simulink model "DigitalTwin_v8"  (R2023a)
settings: Solver=ode23t  StartTime=0.0  StopTime=600  RelTol=1e-3  AbsTol=1e-3
model workspace: external: MATLAB File C:\Users\claud\OneDrive - TUM\COME -TUM\Software lab\Three_wheeled_base\simscape_1\Three_wheeled_base_DataFile1.m (data not in the file)
values from neighbouring files (symbols this model uses):
  brick_pick_global_xy = [brick_pick_global_xy, new_column]    [Three_wheeled_base_DataFile2.m]
  brick_place_global_xy = [brick_place_global_xy, new_column]    [Three_wheeled_base_DataFile2.m]
  platform_destination_mat = [ 1.0 0; 5 0; 0 0; 0 5 ... (first row only)    [Three_wheeled_base_DataFile2.m]
  robotData =     [points_on_pad.mat]
  smiData =     [points_on_pad.mat]    (also in road_points_on_pad.mat)
undefined symbols (not defined in the file or in its folder): X, Y, Z
libraries: sm_lib x246, nesl_utility x86, fl_lib x12, batteryecm_lib x5, ee_lib x3, robotcorelib x1, robotalgslib x1
(part 2 of 8)

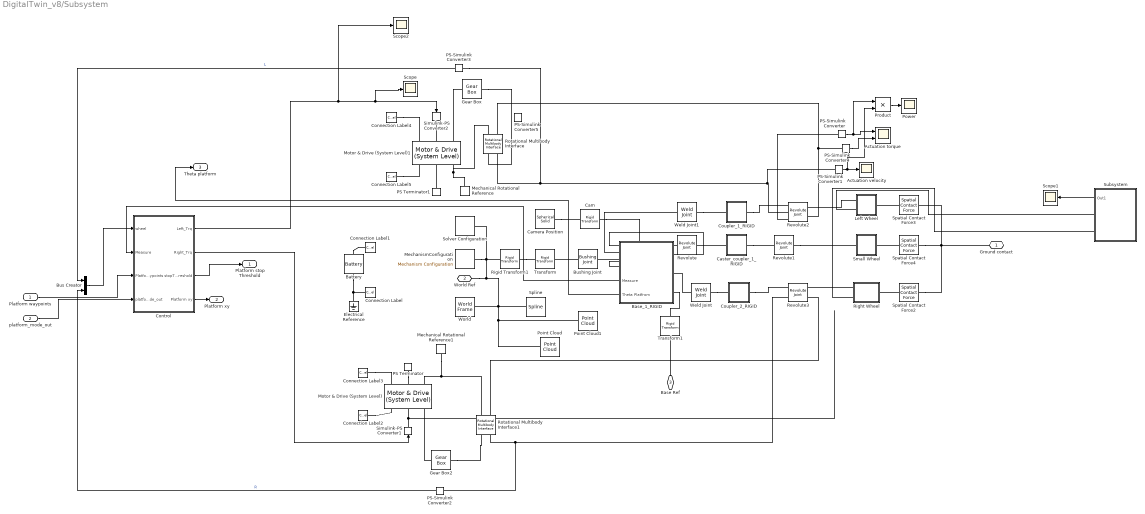
== system DigitalTwin_v8/Subsystem ==
  Platform waypoints : Inport
  platform_mode_out : Inport  Port=2
  Actuation torque : Scope  NumInputPorts=2
  Actuation velocity : Scope
  Base_1_RIGID : Subsystem
      settings: PortSchema="{\"entries\":[{\"content\":{\"sides\":[{\"content\":{\"connectorIds\":[\"LConn1\",\"LConn2\",\"Out1\",\"Out2\"]},\"type\":\"ConnectorPlacement.EquallySpacedRectSide\",\"uuid\":\"915af11b-fe8a-4d36-b5cd-ea91b8047f29\"},{\"content\":{\"connectorIds\":[\"RConn1\",\"RConn2\",\"RConn3\"],\"side\":\"RIGHT\"},\"type\":\"ConnectorPlacement.EquallySpacedRectSide\",\"uuid\":\"f3343107-e0e0-4658-8996-ee38c7783267\"},{\"content\":{\"side\":\"TOP\"},\"type\":\"ConnectorPlacement.EquallySpacedRectSide\",\"uuid\":\"4328f01d-baa2-48a9-97ea-3cbc7b3f5381\"}]},\"type\":\"ConnectorPlacement.EquallySpacedConnector\",\"uuid\":\"91d1c2c9-868d-4769-9f96-4594451c2c0c\"}],\"packageUris\":[\"http://schema.mathworks.com/mf0/Connector/R2020b\"],\"version\":\"1.0\"}"
  Battery : batteryecm_lib/Battery  Vnom=12 V  prm_dir=simscape.enum.battery.prm_dir.disabled  R1_dis=2 Ohm  R1_ch=2 Ohm  R1=2 Ohm  prm_AH=simscape.enum.battery.prm_AH.infinite  AH=50 A*hr  V1=11.5 V  AH1=25 A*hr  prm_R2=simscape.enum.battery.prm_R2.disabled  R2=2000 Ohm  Tmeas=298.15 K  charge_measurement_port=simscape.enum.battery.enable.no  prm_dyn=simscape.enum.battery.prm_dyn.off  Rp1=0.005 Ohm  tau1=30 s  Rp2=0.005 Ohm  tau2=30 s  Rp3=0.005 Ohm  tau3=30 s  Rp4=0.005 Ohm  tau4=30 s  Rp5=0.005 Ohm  tau5=30 s  prm_fade=simscape.enum.battery.prm_fade.disabled  N_fade=100  AH_fade=45 A*hr  R1_fade=2.02 Ohm  R1_ch_fade=2.02 Ohm  V1_fade=10.35 V  prm_age=simscape.enum.battery.prm_age.disabled  prm_age_OCV=simscape.enum.battery.prm_age_OCV.OCV  OCV_age=0.9  SOC_age=60  Tmeas_age=298.15 K  delta_time_age_vec=[0] d  temperature_age_vec=[273] K  OCV_scaling_age=2.2134e6  OCV_offset_age=1.632e6  temp_exp_age=0.515833569 V  t_exp_age=0.75  Vnom_T2=12 V  R1_T2=2.2 Ohm  R1_T2_dis=2.2 Ohm  R1_T2_ch=2.2 Ohm  V1_T2=11.4 V  R2_T2=2200 Ohm  Rp1_T2=0.005 Ohm  tau1_T2=30 s  Rp2_T2=0.005 Ohm  tau2_T2=30 s  Rp3_T2=0.005 Ohm  tau3_T2=30 s  Rp4_T2=0.005 Ohm  tau4_T2=30 s  Rp5_T2=0.005 Ohm  tau5_T2=30 s  Tmeas2=273.15 K  thermal_port=simscape.enum.thermaleffects.omit  thermal_mass=30000 J/K  i_specify=off  i_priority=None  i=0 A  i_nominal_specify=off  i_nominal_unit=A  i_nominal_value=1  v_specify=off  v_priority=None  v=0 V  v_nominal_specify=off  v_nominal_unit=V  v_nominal_value=1  charge_specify=off  charge_priority=High  charge=50 A*hr  charge_nominal_specify=off  charge_nominal_unit=A*hr  charge_nominal_value=1  num_cycles_specify=off  num_cycles_priority=High  num_cycles=0  num_cycles_nominal_specify=off  num_cycles_nominal_unit=1  num_cycles_nominal_value=1  temperature_specify=off  temperature_priority=High  temperature=298.15 K  temperature_nominal_specify=off  temperature_nominal_unit=K  temperature_nominal_value=1
  Bus Creator : BusCreator  Inputs=2
  Bushing Joint : sm_lib/Joints/Bushing Joint  JointMode=Normal  SenseConstraintForce=off  SenseConstraintForceX=off  SenseConstraintForceY=off  SenseConstraintForceZ=off  SenseConstraintTorque=off  SenseConstraintTorqueX=off  SenseConstraintTorqueY=off  SenseConstraintTorqueZ=off  SenseTotalForce=off  SenseTotalForceX=off  SenseTotalForceY=off  SenseTotalForceZ=off  SenseTotalTorque=off  SenseTotalTorqueX=off  SenseTotalTorqueY=off  SenseTotalTorqueZ=off  CompositeWrenchDir=FollowerOnBase  CompositeWrenchFrame=BaseFrame  PxEquilibriumPosition=0  PxEquilibriumPositionUnits=m  PxSpringStiffness=0  PxSpringStiffnessUnits=N/m  PxDampingCoefficient=0  PxDampingCoefficientUnits=N/(m/s)  PxTorqueActuationMode=NoTorque  PxMotionActuationMode=ComputedMotion  PxSensePosition=off  PxSenseVelocity=off  PxSenseAcceleration=off  PxSenseTorqueForce=off  PxSenseLowerLimitTorqueForce=off  PxSenseUpperLimitTorqueForce=off  PxLowerLimitSpecify=off  PxLowerLimitBound=-1  PxLowerLimitBoundUnits=m  PxLowerLimitStiffness=1e6  PxLowerLimitStiffnessUnits=N/m  PxLowerLimitDamping=1e3  PxLowerLimitDampingUnits=N/(m/s)  PxLowerLimitTransitionRegionWidth=1e-4  PxLowerLimitTransitionRegionWidthUnits=m  PxUpperLimitSpecify=off  PxUpperLimitBound=1  PxUpperLimitBoundUnits=m  PxUpperLimitStiffness=1e6  PxUpperLimitStiffnessUnits=N/m  PxUpperLimitDamping=1e3  PxUpperLimitDampingUnits=N/(m/s)  PxUpperLimitTransitionRegionWidth=1e-4  PxUpperLimitTransitionRegionWidthUnits=m  PxPositionTargetSpecify=off  PxPositionTargetPriority=High  PxPositionTargetValue=0  PxPositionTargetValueUnits=m  PxVelocityTargetSpecify=off  PxVelocityTargetPriority=High  PxVelocityTargetValue=0  PxVelocityTargetValueUnits=m/s  PyEquilibriumPosition=0  PyEquilibriumPositionUnits=m  PySpringStiffness=0  PySpringStiffnessUnits=N/m  PyDampingCoefficient=0  PyDampingCoefficientUnits=N/(m/s)  PyTorqueActuationMode=NoTorque  PyMotionActuationMode=ComputedMotion  PySensePosition=off  PySenseVelocity=off  PySenseAcceleration=off  PySenseTorqueForce=off  PySenseLowerLimitTorqueForce=off  PySenseUpperLimitTorqueForce=off  PyLowerLimitSpecify=off  PyLowerLimitBound=-1  PyLowerLimitBoundUnits=m  PyLowerLimitStiffness=1e6  PyLowerLimitStiffnessUnits=N/m  PyLowerLimitDamping=1e3  PyLowerLimitDampingUnits=N/(m/s)  PyLowerLimitTransitionRegionWidth=1e-4  PyLowerLimitTransitionRegionWidthUnits=m  PyUpperLimitSpecify=off  PyUpperLimitBound=1  PyUpperLimitBoundUnits=m  PyUpperLimitStiffness=1e6  PyUpperLimitStiffnessUnits=N/m  PyUpperLimitDamping=1e3  PyUpperLimitDampingUnits=N/(m/s)  PyUpperLimitTransitionRegionWidth=1e-4  PyUpperLimitTransitionRegionWidthUnits=m  PyPositionTargetSpecify=off  PyPositionTargetPriority=High  PyPositionTargetValue=0  PyPositionTargetValueUnits=m  PyVelocityTargetSpecify=off  PyVelocityTargetPriority=High  PyVelocityTargetValue=0  PyVelocityTargetValueUnits=m/s  PzEquilibriumPosition=0  PzEquilibriumPositionUnits=m  PzSpringStiffness=0  PzSpringStiffnessUnits=N/m  PzDampingCoefficient=0  PzDampingCoefficientUnits=N/(m/s)  PzTorqueActuationMode=NoTorque  PzMotionActuationMode=ComputedMotion  PzSensePosition=off  PzSenseVelocity=off  PzSenseAcceleration=off  PzSenseTorqueForce=off  PzSenseLowerLimitTorqueForce=off  PzSenseUpperLimitTorqueForce=off  PzLowerLimitSpecify=off  PzLowerLimitBound=-1  PzLowerLimitBoundUnits=m  PzLowerLimitStiffness=1e6  PzLowerLimitStiffnessUnits=N/m  PzLowerLimitDamping=1e3  PzLowerLimitDampingUnits=N/(m/s)  PzLowerLimitTransitionRegionWidth=1e-4  PzLowerLimitTransitionRegionWidthUnits=m  PzUpperLimitSpecify=off  PzUpperLimitBound=1  PzUpperLimitBoundUnits=m  PzUpperLimitStiffness=1e6  PzUpperLimitStiffnessUnits=N/m  PzUpperLimitDamping=1e3  PzUpperLimitDampingUnits=N/(m/s)  PzUpperLimitTransitionRegionWidth=1e-4  PzUpperLimitTransitionRegionWidthUnits=m  PzPositionTargetSpecify=off  PzPositionTargetPriority=High  PzPositionTargetValue=0  PzPositionTargetValueUnits=m  PzVelocityTargetSpecify=off  PzVelocityTargetPriority=High  PzVelocityTargetValue=0  PzVelocityTargetValueUnits=m/s  RxEquilibriumPosition=0  RxEquilibriumPositionUnits=deg  RxSpringStiffness=0  RxSpringStiffnessUnits=N*m/deg  RxDampingCoefficient=0  RxDampingCoefficientUnits=N*m/(deg/s)  RxTorqueActuationMode=NoTorque  RxMotionActuationMode=ComputedMotion  RxSensePosition=off  RxSenseVelocity=off  RxSenseAcceleration=off  RxSenseTorqueForce=off  RxSenseLowerLimitTorqueForce=off  RxSenseUpperLimitTorqueForce=off  RxLowerLimitSpecify=off  RxLowerLimitBound=-90  RxLowerLimitBoundUnits=deg  RxLowerLimitStiffness=1e4  RxLowerLimitStiffnessUnits=N*m/deg  RxLowerLimitDamping=10  RxLowerLimitDampingUnits=N*m/(deg/s)  RxLowerLimitTransitionRegionWidth=0.1  RxLowerLimitTransitionRegionWidthUnits=deg  RxUpperLimitSpecify=off  RxUpperLimitBound=90  RxUpperLimitBoundUnits=deg  RxUpperLimitStiffness=1e4  RxUpperLimitStiffnessUnits=N*m/deg  RxUpperLimitDamping=10  RxUpperLimitDampingUnits=N*m/(deg/s)  RxUpperLimitTransitionRegionWidth=0.1  RxUpperLimitTransitionRegionWidthUnits=deg  RxPositionTargetSpecify=off  RxPositionTargetPriority=High  RxPositionTargetValue=0  RxPositionTargetValueUnits=deg  RxVelocityTargetSpecify=off  RxVelocityTargetPriority=High  RxVelocityTargetValue=0  RxVelocityTargetValueUnits=deg/s  RyEquilibriumPosition=0  RyEquilibriumPositionUnits=deg  RySpringStiffness=0  RySpringStiffnessUnits=N*m/deg  RyDampingCoefficient=0  RyDampingCoefficientUnits=N*m/(deg/s)  RyTorqueActuationMode=NoTorque  RyMotionActuationMode=ComputedMotion  RySensePosition=off  RySenseVelocity=off  RySenseAcceleration=off  RySenseTorqueForce=off  RySenseLowerLimitTorqueForce=off  RySenseUpperLimitTorqueForce=off  RyLowerLimitSpecify=off  RyLowerLimitBound=-90  RyLowerLimitBoundUnits=deg  RyLowerLimitStiffness=1e4  RyLowerLimitStiffnessUnits=N*m/deg  RyLowerLimitDamping=10  RyLowerLimitDampingUnits=N*m/(deg/s)  RyLowerLimitTransitionRegionWidth=0.1  RyLowerLimitTransitionRegionWidthUnits=deg  RyUpperLimitSpecify=off  RyUpperLimitBound=90  RyUpperLimitBoundUnits=deg  RyUpperLimitStiffness=1e4  RyUpperLimitStiffnessUnits=N*m/deg  RyUpperLimitDamping=10  RyUpperLimitDampingUnits=N*m/(deg/s)  RyUpperLimitTransitionRegionWidth=0.1  RyUpperLimitTransitionRegionWidthUnits=deg  RyPositionTargetSpecify=off  RyPositionTargetPriority=High  RyPositionTargetValue=0  RyPositionTargetValueUnits=deg  RyVelocityTargetSpecify=off  RyVelocityTargetPriority=High  RyVelocityTargetValue=0  RyVelocityTargetValueUnits=deg/s  RzEquilibriumPosition=0  RzEquilibriumPositionUnits=deg  RzSpringStiffness=0  RzSpringStiffnessUnits=N*m/deg  RzDampingCoefficient=0  RzDampingCoefficientUnits=N*m/(deg/s)  RzTorqueActuationMode=NoTorque  RzMotionActuationMode=ComputedMotion  RzSensePosition=off  RzSenseVelocity=off  RzSenseAcceleration=off  RzSenseTorqueForce=off  RzSenseLowerLimitTorqueForce=off  RzSenseUpperLimitTorqueForce=off  RzLowerLimitSpecify=off  RzLowerLimitBound=-90  RzLowerLimitBoundUnits=deg  RzLowerLimitStiffness=1e4  RzLowerLimitStiffnessUnits=N*m/deg  RzLowerLimitDamping=10  RzLowerLimitDampingUnits=N*m/(deg/s)  RzLowerLimitTransitionRegionWidth=0.1  RzLowerLimitTransitionRegionWidthUnits=deg  RzUpperLimitSpecify=off  RzUpperLimitBound=90  RzUpperLimitBoundUnits=deg  RzUpperLimitStiffness=1e4  RzUpperLimitStiffnessUnits=N*m/deg  RzUpperLimitDamping=10  RzUpperLimitDampingUnits=N*m/(deg/s)  RzUpperLimitTransitionRegionWidth=0.1  RzUpperLimitTransitionRegionWidthUnits=deg  RzPositionTargetSpecify=off  RzPositionTargetPriority=High  RzPositionTargetValue=0  RzPositionTargetValueUnits=deg  RzVelocityTargetSpecify=off  RzVelocityTargetPriority=High  RzVelocityTargetValue=0  RzVelocityTargetValueUnits=deg/s
  Cam : sm_lib/Frames and Transforms/Rigid Transform  TranslationMethod=Cartesian  TranslationStandardOffset=0  TranslationStandardOffsetUnits=m  TranslationStandardAxis=+Z  TranslationCartesianOffset=[1 1 1]  TranslationCartesianOffsetUnits=m  TranslationROffset=0  TranslationROffsetUnits=m  TranslationZOffset=0  TranslationZOffsetUnits=m  TranslationThetaOffset=0  TranslationThetaOffsetUnits=deg  RotationMethod=None  RotationAngleUnits=deg  RotationStandardAxis=+Z  RotationAngle=0.0  RotationArbitraryAxis=[0 0 1]  FollAlignAxisA=+X  BaseAlignAxisA=+Y  FollAlignAxisB=+Y  BaseAlignAxisB=+Z  RotationSequenceAxes=FollowerAxes  RotationSequence=XYX  RotationSequenceAngles=[0 0 0]  RotationSequenceAnglesUnits=deg  RotationMatrix=[1 0 0; 0 1 0; 0 0 1]  Quaternion=[1 0 0 0]
  Camera Position : sm_lib/Body Elements/Spherical Solid  GraphicAmbientColor=[0.15 0.15 0.15 1.0]  BasedOnType=Density  CenterOfMass=[0 0 0]  CenterOfMassUnits=m  GraphicDiffuseColor=[0.5 0.5 0.5]  Density=0  DensityUnits=kg/m^3  DoExposeReferenceFrame=on  GraphicEmissiveColor=[0.0 0.0 0.0 1.0]  ExportEntireGeometry=off  SerializedExposedGeometries=<ExposedGeometries/>  SerializedFrames=<Frames/>  MarkerShape=Sphere  MarkerSize=10  GraphicType=FromGeometry  InertiaType=CalculateFromGeometry  Mass=1  MassUnits=kg  MomentsOfInertia=[1 1 1]  MomentsOfInertiaUnits=kg*m^2  GraphicOpacity=1.0  ProductsOfInertia=[0 0 0]  ProductsOfInertiaUnits=kg*m^2  GraphicShininess=75  GraphicSpecularColor=[0.5 0.5 0.5 1.0]  SphereRadius=0.01  SphereRadiusUnits=m  GraphicVisPropType=SimpleVisualProperties
  Caster_coupler_1_RIGID : Subsystem
  Connection Label : ConnectionLabel  Label=N
  Connection Label1 : ConnectionLabel  Label=P
  Connection Label2 : ConnectionLabel  Label=P
  Connection Label3 : ConnectionLabel  Label=N
  Connection Label4 : ConnectionLabel  Label=P
  Connection Label5 : ConnectionLabel  Label=N
  Control : Subsystem
  Coupler_1_RIGID : Subsystem
  Coupler_2_RIGID : Subsystem
  Electrical Reference : fl_lib/Electrical/Electrical Elements/Electrical Reference
  Gear Box : fl_lib/Mechanical/Mechanisms/Gear Box  ratio=0.05*0+1  t_in_specify=off  t_in_priority=None  t_in=0 N*m  t_in_nominal_specify=off  t_in_nominal_unit=N*m  t_in_nominal_value=1  t_out_specify=off  t_out_priority=None  t_out=0 N*m  t_out_nominal_specify=off  t_out_nominal_unit=N*m  t_out_nominal_value=1
  Gear Box2 : fl_lib/Mechanical/Mechanisms/Gear Box  ratio=0.05*0+1  t_in_specify=off  t_in_priority=None  t_in=0 N*m  t_in_nominal_specify=off  t_in_nominal_unit=N*m  t_in_nominal_value=1  t_out_specify=off  t_out_priority=None  t_out=0 N*m  t_out_nominal_specify=off  t_out_nominal_unit=N*m  t_out_nominal_value=1
  Left Wheel : Subsystem
  Mechanical Rotational Reference : fl_lib/Mechanical/Rotational Elements/Mechanical Rotational Reference
  Mechanical Rotational Reference1 : fl_lib/Mechanical/Rotational Elements/Mechanical Rotational Reference
  MechanismConfiguration : sm_lib/Utilities/Mechanism Configuration  UniformGravity=Constant  GravityVector=[0 0 -9.80665]  GravityVectorUnits=m/s^2  LinearizationDelta=0.001  JointModeTransitionNonlinearIterations=2
  Motor & Drive (System Level) : ee_lib/Electromechanical/Motor & Drive (System Level)  torque_speed_param=ee.enum.electromech.envelope.tabulated  overtorque_param=ee.enum.electromech.overtorque.no  T_t=[.09, .08, .07, 0]*20 N*m  T_t_intermittent=[.36, .32, .28, 0] N*m  T_t_2D=[.09, .09, .09; .08, .08, .08; .07, .07, .07; 0, 0, 0] N*m  T_t_intermittent_2D=[.36, .36, .36; .32, .32, .32; .28, .28, .28; 0, 0, 0] N*m  w_t=[0, 3750, 7500, 8000] rpm  vdc_t=[6, 12, 24] V  torque_max=0.1 N*m  power_max=30 W  torque_max_intermittent=0.4 N*m  power_max_intermittent=120 W  time_overtorque=30 s  time_recover=60 s  Tc=0.02 s  losses_param=1  eff=100  w_eff=3750 rpm  T_eff=0.08 N*m  Piron=0 W  Pbase=0 W  w_eff_vec=[-8000, -4000, 0, 4000, 8000] rpm  T_eff_vec=[0, .03, .06, .09] N*m  v_eff_vec=[100, 250, 400] V  losses_mat=[1.49, 1.67, 2.21, 3.1; .42, .69, 1.14, 2.03; .06, .24, .78, 1.68; .42, .69, 1.14, 2.03; 1.49, 1.67, 2.21, 3.1] W  efficiency_mat=[95, 95, 95, 95; 95, 95, 95, 95; 95, 95, 95, 95; 95, 95, 95, 95; 95, 95, 95, 95]  losses_mat_3D=ones(5, 4, 3) W  efficiency_mat_3D=95 * ones(5, 4, 3)  Res=0 Ohm  enable_fault=simscape.enum.onoff.off  fault_condition=1  fault_threshold=0.5  J=5e-6 kg*m^2  lam=1e-5 N*m*s/rad  speed0=0 rpm  faulted_specify=off  faulted_priority=None  faulted=0  faulted_nominal_specify=off  faulted_nominal_unit=1  faulted_nominal_value=1  torqueLimitContinuous_specify=off  torqueLimitContinuous_priority=None  torqueLimitContinuous=0 N*m  torqueLimitContinuous_nominal_specify=off  torqueLimitContinuous_nominal_unit=N*m  torqueLimitContinuous_nominal_value=1  alpha=3.93e-3 1/K  Tmeas=25 degC  Tmeas2=125 degC  losses_mat_T2=[1.49, 1.74, 2.49, 3.74; .42, .67, 1.42, 2.67; .06, .31, 1.06, 2.31; .42, .67, 1.42, 2.67; 1.49, 1.74, 2.49, 3.74] W  efficiency_mat_T2=[95, 95, 95, 95; 95, 95, 95, 95; 95, 95, 95, 95; 95, 95, 95, 95; 95, 95, 95, 95]  losses_mat_3D_T2=ones(5, 4, 3) W  efficiency_mat_3D_T2=95 * ones(5, 4, 3)  thermal_mass=100 J/K  initial_temperature=25 degC
  Motor & Drive (System Level)1 : ee_lib/Electromechanical/Motor & Drive (System Level)  torque_speed_param=ee.enum.electromech.envelope.tabulated  overtorque_param=ee.enum.electromech.overtorque.no  T_t=[.09, .08, .07, 0]*20 N*m  T_t_intermittent=[.36, .32, .28, 0] N*m  T_t_2D=[.09, .09, .09; .08, .08, .08; .07, .07, .07; 0, 0, 0] N*m  T_t_intermittent_2D=[.36, .36, .36; .32, .32, .32; .28, .28, .28; 0, 0, 0] N*m  w_t=[0, 3750, 7500, 8000] rpm  vdc_t=[6, 12, 24] V  torque_max=0.1 N*m  power_max=30 W  torque_max_intermittent=0.4 N*m  power_max_intermittent=120 W  time_overtorque=30 s  time_recover=60 s  Tc=0.02 s  losses_param=1  eff=100  w_eff=3750 rpm  T_eff=0.08 N*m  Piron=0 W  Pbase=0 W  w_eff_vec=[-8000, -4000, 0, 4000, 8000] rpm  T_eff_vec=[0, .03, .06, .09] N*m  v_eff_vec=[100, 250, 400] V  losses_mat=[1.49, 1.67, 2.21, 3.1; .42, .69, 1.14, 2.03; .06, .24, .78, 1.68; .42, .69, 1.14, 2.03; 1.49, 1.67, 2.21, 3.1] W  efficiency_mat=[95, 95, 95, 95; 95, 95, 95, 95; 95, 95, 95, 95; 95, 95, 95, 95; 95, 95, 95, 95]  losses_mat_3D=ones(5, 4, 3) W  efficiency_mat_3D=95 * ones(5, 4, 3)  Res=0 Ohm  enable_fault=simscape.enum.onoff.off  fault_condition=1  fault_threshold=0.5  J=5e-6 kg*m^2  lam=1e-5 N*m*s/rad  speed0=0 rpm  faulted_specify=off  faulted_priority=None  faulted=0  faulted_nominal_specify=off  faulted_nominal_unit=1  faulted_nominal_value=1  torqueLimitContinuous_specify=off  torqueLimitContinuous_priority=None  torqueLimitContinuous=0 N*m  torqueLimitContinuous_nominal_specify=off  torqueLimitContinuous_nominal_unit=N*m  torqueLimitContinuous_nominal_value=1  alpha=3.93e-3 1/K  Tmeas=25 degC  Tmeas2=125 degC  losses_mat_T2=[1.49, 1.74, 2.49, 3.74; .42, .67, 1.42, 2.67; .06, .31, 1.06, 2.31; .42, .67, 1.42, 2.67; 1.49, 1.74, 2.49, 3.74] W  efficiency_mat_T2=[95, 95, 95, 95; 95, 95, 95, 95; 95, 95, 95, 95; 95, 95, 95, 95; 95, 95, 95, 95]  losses_mat_3D_T2=ones(5, 4, 3) W  efficiency_mat_3D_T2=95 * ones(5, 4, 3)  thermal_mass=100 J/K  initial_temperature=25 degC
      settings: LogSimulationData=on
  PS Terminator : fl_lib/Physical Signals/Sinks/PS Terminator
  PS Terminator1 : fl_lib/Physical Signals/Sinks/PS Terminator
  PS-Simulink Converter : nesl_utility/PS-Simulink Converter  PhysicalDomain=network_engine_domain  SubClassName=ps_output  LeftPortType=input  RightPortType=output  PseudoPeriodic=off  Frequencies=[]  VectorFormat=inherit  Unit=N*m  AffineConversion=off
  PS-Simulink Converter1 : nesl_utility/PS-Simulink Converter  PhysicalDomain=network_engine_domain  SubClassName=ps_output  LeftPortType=input  RightPortType=output  PseudoPeriodic=off  Frequencies=[]  VectorFormat=inherit  Unit=rad/s  AffineConversion=off
  PS-Simulink Converter2 : nesl_utility/PS-Simulink Converter  PhysicalDomain=network_engine_domain  SubClassName=ps_output  LeftPortType=input  RightPortType=output  PseudoPeriodic=off  Frequencies=[]  VectorFormat=inherit  Unit=inherit  AffineConversion=off
  PS-Simulink Converter3 : nesl_utility/PS-Simulink Converter  PhysicalDomain=network_engine_domain  SubClassName=ps_output  LeftPortType=input  RightPortType=output  PseudoPeriodic=off  Frequencies=[]  VectorFormat=inherit  Unit=inherit  AffineConversion=off
  PS-Simulink Converter4 : nesl_utility/PS-Simulink Converter  PhysicalDomain=network_engine_domain  SubClassName=ps_output  LeftPortType=input  RightPortType=output  PseudoPeriodic=off  Frequencies=[]  VectorFormat=inherit  Unit=N*m  AffineConversion=off
  PS-Simulink Converter5 : nesl_utility/PS-Simulink Converter  PhysicalDomain=network_engine_domain  SubClassName=ps_output  LeftPortType=input  RightPortType=output  PseudoPeriodic=off  Frequencies=[]  VectorFormat=inherit  Unit=inherit  AffineConversion=off
  Point Cloud : sm_lib/Curves and Surfaces/Point Cloud  CoordinatesMatrix=plotPoint_mtx  CoordinatesMatrixUnits=m  GraphicType=MarkerCloud  GraphicSphereRadius=1e-1  GraphicSphereRadiusUnits=m  GraphicVisPropType=SimpleVisualProperties  GraphicDiffuseColor=[1 0 1]  GraphicOpacity=1.0  GraphicSpecularColor=[0.5 0.5 0.5 1.0]  GraphicAmbientColor=[0.15 0.15 0.15 1.0]  GraphicEmissiveColor=[0.0 0.0 0.0 1.0]  GraphicShininess=75
  Point Cloud1 : sm_lib/Curves and Surfaces/Point Cloud  CoordinatesMatrix="[0.0253598785439431\t4.98644041888993\t1.45178955108506;-0.00960382399913822\t5.59952231514609\t0.175377640503004;-0.00940823618023848\t5.60012137569571\t0.399787372013566]"  CoordinatesMatrixUnits=m  GraphicType=MarkerCloud  GraphicSphereRadius=2.5e-2  GraphicSphereRadiusUnits=m  GraphicVisPropType=SimpleVisualProperties  GraphicDiffuseColor=[0.851 0.3255 0.09804]  GraphicOpacity=1.0  GraphicSpecularColor=[0.5 0.5 0.5 1.0]  GraphicAmbientColor=[0.15 0.15 0.15 1.0]  GraphicEmissiveColor=[0.0 0.0 0.0 1.0]  GraphicShininess=75
  Power : Scope
  Product : Product
  Revolute : sm_lib/Joints/Revolute Joint  JointMode=Normal  SenseConstraintForce=off  SenseConstraintForceX=off  SenseConstraintForceY=off  SenseConstraintForceZ=off  SenseConstraintTorque=off  SenseConstraintTorqueX=off  SenseConstraintTorqueY=off  SenseConstraintTorqueZ=off  SenseTotalForce=off  SenseTotalForceX=off  SenseTotalForceY=off  SenseTotalForceZ=off  SenseTotalTorque=off  SenseTotalTorqueX=off  SenseTotalTorqueY=off  SenseTotalTorqueZ=off  CompositeWrenchDir=FollowerOnBase  CompositeWrenchFrame=BaseFrame  EquilibriumPosition=0  EquilibriumPositionUnits=deg  SpringStiffness=0  SpringStiffnessUnits=N*m/deg  DampingCoefficient=0  DampingCoefficientUnits=N*m/(deg/s)  TorqueActuationMode=NoTorque  MotionActuationMode=ComputedMotion  SensePosition=off  SenseVelocity=off  SenseAcceleration=off  SenseTorqueForce=off  SenseLowerLimitTorqueForce=off  SenseUpperLimitTorqueForce=off  LowerLimitSpecify=off  LowerLimitBound=-90  LowerLimitBoundUnits=deg  LowerLimitStiffness=1e4  LowerLimitStiffnessUnits=N*m/deg  LowerLimitDamping=10  LowerLimitDampingUnits=N*m/(deg/s)  LowerLimitTransitionRegionWidth=0.1  LowerLimitTransitionRegionWidthUnits=deg  UpperLimitSpecify=off  UpperLimitBound=90  UpperLimitBoundUnits=deg  UpperLimitStiffness=1e4  UpperLimitStiffnessUnits=N*m/deg  UpperLimitDamping=10  UpperLimitDampingUnits=N*m/(deg/s)  UpperLimitTransitionRegionWidth=0.1  UpperLimitTransitionRegionWidthUnits=deg  PositionTargetSpecify=on  PositionTargetPriority=Low  PositionTargetValue=smiData.RevoluteJoint(1).Rz.Pos  PositionTargetValueUnits=deg  VelocityTargetSpecify=off  VelocityTargetPriority=High  VelocityTargetValue=0  VelocityTargetValueUnits=deg/s
  Revolute1 : sm_lib/Joints/Revolute Joint  JointMode=Normal  SenseConstraintForce=off  SenseConstraintForceX=off  SenseConstraintForceY=off  SenseConstraintForceZ=off  SenseConstraintTorque=off  SenseConstraintTorqueX=off  SenseConstraintTorqueY=off  SenseConstraintTorqueZ=off  SenseTotalForce=off  SenseTotalForceX=off  SenseTotalForceY=off  SenseTotalForceZ=off  SenseTotalTorque=off  SenseTotalTorqueX=off  SenseTotalTorqueY=off  SenseTotalTorqueZ=off  CompositeWrenchDir=FollowerOnBase  CompositeWrenchFrame=BaseFrame  EquilibriumPosition=0  EquilibriumPositionUnits=deg  SpringStiffness=0  SpringStiffnessUnits=N*m/deg  DampingCoefficient=0  DampingCoefficientUnits=N*m/(deg/s)  TorqueActuationMode=NoTorque  MotionActuationMode=ComputedMotion  SensePosition=off  SenseVelocity=off  SenseAcceleration=off  SenseTorqueForce=off  SenseLowerLimitTorqueForce=off  SenseUpperLimitTorqueForce=off  LowerLimitSpecify=off  LowerLimitBound=-90  LowerLimitBoundUnits=deg  LowerLimitStiffness=1e4  LowerLimitStiffnessUnits=N*m/deg  LowerLimitDamping=10  LowerLimitDampingUnits=N*m/(deg/s)  LowerLimitTransitionRegionWidth=0.1  LowerLimitTransitionRegionWidthUnits=deg  UpperLimitSpecify=off  UpperLimitBound=90  UpperLimitBoundUnits=deg  UpperLimitStiffness=1e4  UpperLimitStiffnessUnits=N*m/deg  UpperLimitDamping=10  UpperLimitDampingUnits=N*m/(deg/s)  UpperLimitTransitionRegionWidth=0.1  UpperLimitTransitionRegionWidthUnits=deg  PositionTargetSpecify=on  PositionTargetPriority=Low  PositionTargetValue=smiData.RevoluteJoint(2).Rz.Pos  PositionTargetValueUnits=deg  VelocityTargetSpecify=off  VelocityTargetPriority=High  VelocityTargetValue=0  VelocityTargetValueUnits=deg/s
  Revolute2 : sm_lib/Joints/Revolute Joint  JointMode=Normal  SenseConstraintForce=off  SenseConstraintForceX=off  SenseConstraintForceY=off  SenseConstraintForceZ=off  SenseConstraintTorque=off  SenseConstraintTorqueX=off  SenseConstraintTorqueY=off  SenseConstraintTorqueZ=off  SenseTotalForce=off  SenseTotalForceX=off  SenseTotalForceY=off  SenseTotalForceZ=off  SenseTotalTorque=off  SenseTotalTorqueX=off  SenseTotalTorqueY=off  SenseTotalTorqueZ=off  CompositeWrenchDir=FollowerOnBase  CompositeWrenchFrame=BaseFrame  EquilibriumPosition=0  EquilibriumPositionUnits=deg  SpringStiffness=0  SpringStiffnessUnits=N*m/deg  DampingCoefficient=0.001  DampingCoefficientUnits=N*m/(deg/s)  TorqueActuationMode=InputTorque  MotionActuationMode=ComputedMotion  SensePosition=off  SenseVelocity=on  SenseAcceleration=off  SenseTorqueForce=on  SenseLowerLimitTorqueForce=off  SenseUpperLimitTorqueForce=off  LowerLimitSpecify=off  LowerLimitBound=-90  LowerLimitBoundUnits=deg  LowerLimitStiffness=1e4  LowerLimitStiffnessUnits=N*m/deg  LowerLimitDamping=10  LowerLimitDampingUnits=N*m/(deg/s)  LowerLimitTransitionRegionWidth=0.1  LowerLimitTransitionRegionWidthUnits=deg  UpperLimitSpecify=off  UpperLimitBound=90  UpperLimitBoundUnits=deg  UpperLimitStiffness=1e4  UpperLimitStiffnessUnits=N*m/deg  UpperLimitDamping=10  UpperLimitDampingUnits=N*m/(deg/s)  UpperLimitTransitionRegionWidth=0.1  UpperLimitTransitionRegionWidthUnits=deg  PositionTargetSpecify=on  PositionTargetPriority=Low  PositionTargetValue=smiData.RevoluteJoint(3).Rz.Pos  PositionTargetValueUnits=deg  VelocityTargetSpecify=off  VelocityTargetPriority=High  VelocityTargetValue=0  VelocityTargetValueUnits=deg/s
  Revolute3 : sm_lib/Joints/Revolute Joint  JointMode=Normal  SenseConstraintForce=off  SenseConstraintForceX=off  SenseConstraintForceY=off  SenseConstraintForceZ=off  SenseConstraintTorque=off  SenseConstraintTorqueX=off  SenseConstraintTorqueY=off  SenseConstraintTorqueZ=off  SenseTotalForce=off  SenseTotalForceX=off  SenseTotalForceY=off  SenseTotalForceZ=off  SenseTotalTorque=off  SenseTotalTorqueX=off  SenseTotalTorqueY=off  SenseTotalTorqueZ=off  CompositeWrenchDir=FollowerOnBase  CompositeWrenchFrame=BaseFrame  EquilibriumPosition=0  EquilibriumPositionUnits=deg  SpringStiffness=0  SpringStiffnessUnits=N*m/deg  DampingCoefficient=0.001  DampingCoefficientUnits=N*m/(deg/s)  TorqueActuationMode=InputTorque  MotionActuationMode=ComputedMotion  SensePosition=off  SenseVelocity=on  SenseAcceleration=off  SenseTorqueForce=off  SenseLowerLimitTorqueForce=off  SenseUpperLimitTorqueForce=off  LowerLimitSpecify=off  LowerLimitBound=-90  LowerLimitBoundUnits=deg  LowerLimitStiffness=1e4  LowerLimitStiffnessUnits=N*m/deg  LowerLimitDamping=10  LowerLimitDampingUnits=N*m/(deg/s)  LowerLimitTransitionRegionWidth=0.1  LowerLimitTransitionRegionWidthUnits=deg  UpperLimitSpecify=off  UpperLimitBound=90  UpperLimitBoundUnits=deg  UpperLimitStiffness=1e4  UpperLimitStiffnessUnits=N*m/deg  UpperLimitDamping=10  UpperLimitDampingUnits=N*m/(deg/s)  UpperLimitTransitionRegionWidth=0.1  UpperLimitTransitionRegionWidthUnits=deg  PositionTargetSpecify=on  PositionTargetPriority=Low  PositionTargetValue=smiData.RevoluteJoint(4).Rz.Pos  PositionTargetValueUnits=deg  VelocityTargetSpecify=off  VelocityTargetPriority=High  VelocityTargetValue=0  VelocityTargetValueUnits=deg/s
  Right Wheel : Subsystem
  Rigid Transform1 : sm_lib/Frames and Transforms/Rigid Transform  TranslationMethod=Cartesian  TranslationStandardOffset=0  TranslationStandardOffsetUnits=m  TranslationStandardAxis=+Z  TranslationCartesianOffset=[0 0 0.1]  TranslationCartesianOffsetUnits=m  TranslationROffset=0  TranslationROffsetUnits=m  TranslationZOffset=0  TranslationZOffsetUnits=m  TranslationThetaOffset=0  TranslationThetaOffsetUnits=deg  RotationMethod=StandardAxis  RotationAngleUnits=deg  RotationStandardAxis=+X  RotationAngle=90.0  RotationArbitraryAxis=[0 0 1]  FollAlignAxisA=+X  BaseAlignAxisA=+Y  FollAlignAxisB=+Y  BaseAlignAxisB=+Z  RotationSequenceAxes=FollowerAxes  RotationSequence=XYX  RotationSequenceAngles=[0 0 0]  RotationSequenceAnglesUnits=deg  RotationMatrix=[1 0 0; 0 1 0; 0 0 1]  Quaternion=[1 0 0 0]
  Rotational Multibody Interface : fl_lib/Mechanical/Multibody Interfaces/Rotational Multibody Interface
  Rotational Multibody Interface1 : fl_lib/Mechanical/Multibody Interfaces/Rotational Multibody Interface
  Scope : Scope
  Scope1 : Scope
  Scope2 : Scope
  Simulink-PS Converter1 : nesl_utility/Simulink-PS Converter  PhysicalDomain=network_engine_domain  SubClassName=ps_input  LeftPortType=input  RightPortType=output  PseudoPeriodic=off  Frequencies=[]  NoiseDistribution=none  NoiseParameters=[]  Unit=1  AffineConversion=off  FilteringAndDerivatives=provide  SimscapeFilterOrder=1  InputFilterTimeConstant=0.001  UdotUserProvided=0
  Simulink-PS Converter2 : nesl_utility/Simulink-PS Converter  PhysicalDomain=network_engine_domain  SubClassName=ps_input  LeftPortType=input  RightPortType=output  PseudoPeriodic=off  Frequencies=[]  NoiseDistribution=none  NoiseParameters=[]  Unit=1  AffineConversion=off  FilteringAndDerivatives=provide  SimscapeFilterOrder=1  InputFilterTimeConstant=0.001  UdotUserProvided=0
  Small Wheel : Subsystem
  Solver Configuration : nesl_utility/Solver Configuration  PhysicalDomain=network_engine_domain  SubClassName=solver  LeftPortType=input  RightPortType=generic  Tones=[]  Harmonics=[]  SimulateNoise=off  Profile=off  UseLocalSampling=off  EnableSwitchedLinearOptims=on  FrequencyDomain=off  UseCCode=off  RelTol=0.001  AbsTol=0.001  MinStep=1e-09  ToWorkspace=off  RevertToSquareIcSolve=off  NumHomotopyIterations=100  PhasorMode=off  PhasorModeNumHarmonics=1  ConsistencySolver=NEWTON_XTOL_AFTER_FTOL  IndexReductionMethod=DerivativeReplacement  DoDC=off  ResidualTolerance=1e-09  ConsistencyTolSource=GLOBAL  ConsistencyAbsTol=0.001  ConsistencyRelTol=0.001  ConsistencyTolFactor=0.001  UseLocalSolver=off  LocalSolverChoice=NE_BACKWARD_EULER_ADVANCER  ResolveIndetEquations=on  FunctionEvalNumThread=1  LocalSolverSampleTime=0.001  DoFixedCost=off  MaxNonlinIter=3  MaxModeIter=2  ComputeImpulses=off  ImpulseIterations=2  LinearAlgebra=auto  LinearAlgebraNumThread=0  EquationFormulation=NE_TIME_EF  DelaysMemoryBudget=1024  AutomaticFiltering=on  FilteringTimeConstant=0.001  PartitionStorageMethod=AS_NEEDED  PartitionMemoryBudget=1024  PartitionMethod=ROBUST
  Spatial Contact Force2 : sm_lib/Forces and Torques/Spatial Contact Force  SenseContactBaseRotation=off  SenseContactBaseTranslation=off  CoefficientOfDynamicFriction=0.7  CoefficientOfStaticFriction=0.9  NormalDamping=10000  NormalDampingUnits=N/(m/s)  SenseContactSignal=off  NormalStiffness=1000000  NormalStiffnessUnits=N/m  FrictionalCriticalVelocity=1e-2  FrictionalCriticalVelocityUnits=m/s  ZeroCrossDetectContactStartAndEnd=off  SenseContactFollowerRotation=off  SenseContactFollowerTranslation=off  FrictionType=SmoothStickSlip  SenseFrictionalForceMagnitude=off  SenseNormalForceMagnitude=off  NormalForceType=SmoothSpringDamper  SenseNormalVelocity=off  SenseSeparationDistance=off  SenseTangentialVelocity=off  NormalTransitionRegionWidth=0.3  NormalTransitionRegionWidthUnits=m
  Spatial Contact Force3 : sm_lib/Forces and Torques/Spatial Contact Force  SenseContactBaseRotation=off  SenseContactBaseTranslation=off  CoefficientOfDynamicFriction=0.7  CoefficientOfStaticFriction=0.9  NormalDamping=10000  NormalDampingUnits=N/(m/s)  SenseContactSignal=off  NormalStiffness=1000000  NormalStiffnessUnits=N/m  FrictionalCriticalVelocity=1e-2  FrictionalCriticalVelocityUnits=m/s  ZeroCrossDetectContactStartAndEnd=off  SenseContactFollowerRotation=off  SenseContactFollowerTranslation=off  FrictionType=SmoothStickSlip  SenseFrictionalForceMagnitude=off  SenseNormalForceMagnitude=off  NormalForceType=SmoothSpringDamper  SenseNormalVelocity=off  SenseSeparationDistance=off  SenseTangentialVelocity=off  NormalTransitionRegionWidth=0.3  NormalTransitionRegionWidthUnits=m
  Spatial Contact Force4 : sm_lib/Forces and Torques/Spatial Contact Force  SenseContactBaseRotation=off  SenseContactBaseTranslation=off  CoefficientOfDynamicFriction=0.7  CoefficientOfStaticFriction=0.9  NormalDamping=10000  NormalDampingUnits=N/(m/s)  SenseContactSignal=off  NormalStiffness=2000000  NormalStiffnessUnits=N/m  FrictionalCriticalVelocity=1e-2  FrictionalCriticalVelocityUnits=m/s  ZeroCrossDetectContactStartAndEnd=off  SenseContactFollowerRotation=off  SenseContactFollowerTranslation=off  FrictionType=SmoothStickSlip  SenseFrictionalForceMagnitude=off  SenseNormalForceMagnitude=off  NormalForceType=SmoothSpringDamper  SenseNormalVelocity=off  SenseSeparationDistance=off  SenseTangentialVelocity=off  NormalTransitionRegionWidth=0.3  NormalTransitionRegionWidthUnits=m
  Spline : sm_lib/Curves and Surfaces/Spline  GraphicAmbientColor=[0.15 0.15 0.15 1.0]  GraphicDiffuseColor=[0.0 0.2 0.8]  DataPoints=|  DataPointsUnits=m  GraphicEmissiveColor=[0.0 0.0 0.0 1.0]  EndConditionType=Natural  MarkerShape=Cube  MarkerSize=10  GraphicType=FromGeometry  GraphicOpacity=1.0  GraphicShininess=75  GraphicSpecularColor=[0.5 0.5 0.5 1.0]  GraphicVisPropType=SimpleVisualProperties
      | [0.0253598785439431	4.98644041888993	1.45178955108506
      | 0.0253580588709075	4.98680548441364	1.45178931588981
      | 0.0253555112127364	4.98726465647309	1.45178700818111
      | 0.0253525667220862	4.98779415967058	1.45178115592038
      | 0.0253505046875558	4.98838687734835	1.45177198000947
      | 0.0253521089403995	4.98903598385673	1.45176110076862
      | 0.0253572823456598	4.98937866756933	1.45175721945251
      | 0.0253578305766444	4.98939853172921	1.45175715696325
      | 0.0253579641911327	4.98940309791654	1.45175714812860
      | 0.0253581142895397	4.98940810914254	1.45175714126109
      | 0.0253594230745629	4.98944699163920	1.45175720878718
      | 0.0253621981030991	4.98950595090739	1.45175799387708
      | 0.0253713939861187	4.98954885140558	1.45176507355250
      | 0.0253844910045290	4.98929775401342	1.45178474633263
      | 0.0253925091912901	4.98859738616365	1.45181166974330
      | 0.0253838255201913	4.98791808041699	1.45182106894271
      | 0.0253627433770685	4.98765123949999	1.45181659448694
      | 0.0253304198473426	4.98833291080799	1.45181462758984
      | 0.0253154033709718	4.99041903723731	1.45181571471392
      | 0.0253318327772921	4.99319213678405	1.45178600089223
      | 0.0253906470103094	4.99708997649823	1.45172622854391
      | 0.0254810021076592	5.00208721280135	1.45168588209834
      | 0.0255271062396158	5.00639625673915	1.45159799324606
      | 0.0255857928712776	5.01242366553454	1.45142909971586
      | 0.0257341961475754	5.02033395486886	1.45116756950288
      | 0.0260087217035412	5.02921266713725	1.45076259677950
      | 0.0265860844627540	5.04305178685665	1.44997080914243
      | 0.0271485840689656	5.05461021936248	1.44910852171124
      | 0.0282515757407400	5.07315167717939	1.44741768758157
      | 0.0298501971206063	5.09386180616036	1.44502422760047
      | 0.0322589859639649	5.11909176826545	1.44140314973867
      | 0.0364473955737421	5.15489853124863	1.43490812811008
      | 0.0431333838410757	5.20074868496064	1.42420993127532
      | 0.0474966478756713	5.22663337409383	1.41695839976729
      | 0.0578466910693974	5.28084640967813	1.39880546053737
      | 0.0642494169610320	5.31106262822849	1.38687558951489
      | 0.0779121358864200	5.37048221712917	1.35934236310501
      | 0.0869475245284388	5.40729421099867	1.33939340250204
      | 0.0935157085932867	5.43324542927550	1.32388248604091
      | 0.0948784210816465	5.43856675285338	1.32054944287714
      | 0.0970883813566028	5.44718762441413	1.31504663228912
      | 0.103231287588324	5.47102496009994	1.29913437451387
      | 0.108612505886898	5.49160100579174	1.28447999122448
      | 0.115895613859323	5.51904223478832	1.26337778156429
      | 0.122670673135640	5.54455006883028	1.24204210125099
      | 0.130879072455982	5.57592654729132	1.21351487740153
      | 0.138284982217049	5.60477718550750	1.18478947857472
      | 0.148028773353476	5.64381417982526	1.14128505081210
      | 0.155683334682769	5.67633233443055	1.10012872773772
      | 0.163976836448669	5.71541329115834	1.04322881604000
      | 0.170072145603857	5.75008664796678	0.983267436429234
      | 0.171879617161309	5.76299329824726	0.957813217093940
      | 0.173126270773318	5.77379064117976	0.934809139135929
      | 0.174438124395523	5.79065825259883	0.894885082399548
      | 0.174701228338848	5.80450479443380	0.857119015013214
      | 0.173331916895375	5.82162717202767	0.800335695225606
      | 0.171720084095070	5.82906228149316	0.769736270969529
      | 0.168603686314391	5.83707039970602	0.728807572302717
      | 0.164417244640424	5.84281856434723	0.688239873754111
      | 0.159199234223326	5.84632889478266	0.648243342257558
      | 0.153265200134140	5.84762934662773	0.610566279682360
      | 0.146215318475671	5.84688601283134	0.572425191764206
      | 0.133361783939709	5.84152218579299	0.514373702990094
      | 0.120534350571409	5.83275523338296	0.465955416656423
      | 0.108615906188523	5.82241163440006	0.426766494307800
      | 0.100633245900991	5.81450907956322	0.402916412784840
      | 0.0993910191653570	5.81321571036993	0.399354028776519
      | 0.0989145944353896	5.81271624554283	0.397997270460255
      | 0.0973474440226019	5.81105928788268	0.393569636025290
      | 0.0944745010846697	5.80796114496756	0.385591179857058
      | 0.0901972429749011	5.80319149004364	0.374064402661472
      | 0.0859599992745633	5.79827722603401	0.363093259965227
      | 0.0802023896338287	5.79129011122882	0.348825660689140
      | 0.0745690353280031	5.78412116196053	0.335420333121322
      | 0.0682598027549659	5.77572197510924	0.320951717185005
      | 0.0598327118139095	5.76385126113159	0.302554722274834
      | 0.0535218551133430	5.75441896524991	0.289433370118120
      | 0.0475369177751226	5.74501655785813	0.277422549245101
      | 0.0382275652517824	5.72941387039021	0.259555637629718
      | 0.0289406428134638	5.71243501938339	0.242592835814602
      | 0.0209714528090902	5.69644893204210	0.228637888390683
      | 0.0127999896320958	5.67823809226492	0.214760176112212
      | 0.00943475906255616	5.67002556389832	0.209138354367628
      | 0.00450838058090862	5.65699156723437	0.200928682023927
      | -0.000293158890293846	5.64268926212230	0.192866971299527
      | -0.00410065128879357	5.62962579502042	0.186288254936027
      | -0.00705221798045553	5.61773307685142	0.180887538042638
      | -0.00865704490086786	5.61010413275333	0.177696197243810
      | -0.00977588442871484	5.60375548146062	0.175197512025912
      | -0.0100868106222834	5.60156720093120	0.174373140932688
      | -0.0102362980598269	5.59998662364369	0.173786632744429
      | -0.0102322119378371	5.59979638466040	0.173719243212255
      | -0.0102174115664225	5.59971670178611	0.173692308420145
      | -0.0102046387370728	5.59969578010306	0.173685892996299
      | -0.0101990447743611	5.59969242342514	0.173685110458489
      | -0.0101968272373785	5.59969179122821	0.173685043669212
      | -0.0101963854870715	5.59969170646695	0.173685045045353
      | -0.0101947425011854	5.59969140456398	0.173685085231522
      | -0.0101909022818816	5.59969073239577	0.173685390635665
      | -0.0101870936345306	5.59969011140140	0.173685985982043
      | -0.0101831107951457	5.59968950753765	0.173686918734292
      | -0.0101788265747718	5.59968890504625	0.173688274323176
      | -0.0101572185360420	5.59968633278472	0.173700653624863
      | -0.0101402729479509	5.59968415368209	0.173716588047851
      | -0.0101291216017233	5.59968193834690	0.173725038485008
      | -0.0101197777208454	5.59968012279836	0.173719706823127
      | -0.0101123540288928	5.59967995804670	0.173706243798099
      | -0.0101116936344798	5.59968003580784	0.173704855957228
      | -0.0101116377808275	5.59968004319366	0.173704738689285
      | -0.0101113341434776	5.59968008551836	0.173704102219767
      | -0.0101106292575028	5.59968019805932	0.173702636608902
      | -0.0101094158694951	5.59968043828115	0.173700191993935
      | -0.0101040794417476	5.59968199383909	0.173692552872821
      | -0.0100979500632790	5.59968381088590	0.173692108904483
      | -0.0100917496731244	5.59968488426095	0.173697456874507
      | -0.0100747110286779	5.59968386053194	0.173712265722229
      | -0.0100535004632871	5.59968189164408	0.173700617908111
      | -0.0100318748715030	5.59968296795190	0.173703296934892
      | -0.0100013903174336	5.59968173135949	0.173703713791694
      | -0.00998668972048371	5.59968176433064	0.173700168993979
      | -0.00997826160116561	5.59968200741265	0.173703264914021
      | -0.00996847420317802	5.59968191992992	0.173707608231428
      | -0.00996049891292660	5.59968149756989	0.173708226727207
      | -0.00995426206186046	5.59968110632075	0.173706460321841
      | -0.00995240812480719	5.59968100793244	0.173705701255074
      | -0.00995182403584412	5.59968097995770	0.173705453129450
      | -0.00995168318151223	5.59968097345021	0.173705392961401
      | -0.00995161062877246	5.59968097013543	0.173705361934616
      | -0.00995137191061253	5.59968095940959	0.173705259722127
      | -0.00995130888981482	5.59968095662472	0.173705232714288
      | -0.00995118712500438	5.59968095129988	0.173705180514545
      | -0.00995105809342435	5.59968094573833	0.173705125187305
      | -0.00995062999314807	5.59968092789374	0.173704941727026
      | -0.00994409144403709	5.59968078024300	0.173702537056372
      | -0.00991697089886614	5.59968100189317	0.173706548259818
      | -0.00988014246580958	5.59968007437299	0.173702865457513
      | -0.00985975873417633	5.59967993027326	0.173707068696886
      | -0.00984762433551086	5.59967935921997	0.173706390462009
      | -0.00982849768145285	5.59967901592197	0.173704344040998
      | -0.00979840748089612	5.59967851598844	0.173706214637288
      | -0.00977345864078321	5.59967813636007	0.173705328844091
      | -0.00976195477020151	5.59967795811140	0.173706526320709
      | -0.00975938701080797	5.59967788879507	0.173706582389909
      | -0.00975835073861000	5.59967785877898	0.173706573799917
      | -0.00975808114057668	5.59967785082664	0.173706568675675
      | -0.00975795855865121	5.59967784719397	0.173706565957912
      | -0.00975792613262811	5.59967784623136	0.173706565198688
      | -0.00975791293612373	5.59967784583940	0.173706564884890
      | -0.00975790698423108	5.59967784566259	0.173706564742450
      | -0.00975790657244529	5.59967784565035	0.173706564732574
      | -0.00975790631587013	5.59967784564273	0.173706564726419
      | -0.00975787970687249	5.59967784485185	0.173706564079695
      | -0.00975733726099657	5.59967782861136	0.173706547134654
      | -0.00975658925640239	5.59967780604501	0.173706510930412
      | -0.00975584135419967	5.59967778352630	0.173706459121240
      | -0.00975434617858165	5.59967773926948	0.173706311334940
      | -0.00973201685090241	5.59967752931987	0.173704009827806
      | -0.00973186338450035	5.59967749074777	0.173705326253826
      | -0.00973409028607444	5.59967661810912	0.173732917435903
      | -0.00974398774119089	5.59967264895086	0.173844243918203
      | -0.00975735494803475	5.59966174748278	0.174082102188872
      | -0.00975819141622594	5.59966023426431	0.174109993046890
      | -0.00975825458717033	5.59966010477672	0.174112334380514
      | -0.00975825870572126	5.59966009624255	0.174112488461163
      | -0.00975828026276841	5.59966005137886	0.174113298359584
      | -0.00975844383614488	5.59965969966569	0.174119642088343
      | -0.00975926627432265	5.59965745748407	0.174159805967490
      | -0.00975950528750741	5.59965004486118	0.174287727428931
      | -0.00975337271139848	5.59963780635373	0.174478175199093
      | -0.00973806382240674	5.59962194826496	0.174686683063930
      | -0.00970951192066456	5.59959868742936	0.174928865388725
      | -0.00967639693069527	5.59957193575192	0.175137407284347
      | -0.00964092373652529	5.59953690988837	0.175326330988061
      | -0.00962886287887224	5.59952039713813	0.175386640708382
      | -0.00962264690176217	5.59950916078270	0.175416264067378
      | -0.00962174510765118	5.59950723439865	0.175420179619029
      | -0.00962159714091122	5.59950690890693	0.175420799939315
      | -0.00962155795036079	5.59950682224165	0.175420962983451
      | -0.00962151054352281	5.59950671715130	0.175421159477765
      | -0.00962145907773302	5.59950660274561	0.175421371865637
      | -0.00962139570380473	5.59950646141375	0.175421632025507
      | -0.00962135965164186	5.59950638078840	0.175421779331539
      | -0.00962132191911238	5.59950629623069	0.175421932950824
      | -0.00962128086897659	5.59950620403552	0.175422099421306
      | -0.00962127055275204	5.59950618083291	0.175422141147435
      | -0.00962126652347170	5.59950617176687	0.175422157432663
      | -0.00962126443988901	5.59950616707793	0.175422165851263
      | -0.00962126220623571	5.59950616205067	0.175422174874198
      | -0.00962125430742466	5.59950614426785	0.175422206764988
      | -0.00962121545054138	5.59950605667436	0.175422363261904
      | -0.00962111903819169	5.59950583851861	0.175422748728829
      | -0.00962105174185636	5.59950568555501	0.175423015297383
      | -0.00962103850772017	5.59950565540742	0.175423067470268
      | -0.00962100824325291	5.59950558638233	0.175423186467497
      | -0.00962095619968174	5.59950546741836	0.175423390056589
      | -0.00962092262197244	5.59950539048612	0.175423520694109
      | -0.00962091626331892	5.59950537590163	0.175423545368807
      | -0.00962090457696655	5.59950534908424	0.175423590663656
      | -0.00962089194743817	5.59950532008351	0.175423639535122
      | -0.00962088756060215	5.59950531000557	0.175423656491189
      | -0.00962088231722419	5.59950529795676	0.175423676744858
      | -0.00962085277490514	5.59950523000788	0.175423790589220
      | -0.00962080408260273	5.59950511777901	0.175423977215692
      | -0.00962079414128720	5.59950509482997	0.175424015160554
      | -0.00962078819578572	5.59950508109930	0.175424037827929
      | -0.00962076489560861	5.59950502724781	0.175424126471966
      | -0.00962066131673811	5.59950478706006	0.175424516797757
      | -0.00962045654110180	5.59950430846380	0.175425269276960
      | -0.00962039039012923	5.59950415282350	0.175425506476540
      | -0.00962032419136825	5.59950399658335	0.175425740764306
      | -0.00962014322343132	5.59950356708966	0.175426364411489
      | -0.00961992215245131	5.59950303809524	0.175427089248141
      | -0.00961970130326098	5.59950250568415	0.175427766734431
      | -0.00961803033165869	5.59949862652653	0.175430388935395
      | -0.00961624593660518	5.59949698107490	0.175424202733152
      | -0.00961600419488815	5.59949712898076	0.175422713357525
      | -0.00961583251478050	5.59949727963446	0.175421628062507
      | -0.00961574759585849	5.59949736658449	0.175421086761397
      | -0.00961558429514845	5.59949755451078	0.175420042719875
      | -0.00961531917214679	5.59949791003441	0.175418352922635
      | -0.00961491102303551	5.59949855322119	0.175415803039127
      | -0.00961464103245562	5.59949902673640	0.175414168124451
      | -0.00961440926734243	5.59949945618212	0.175412803480247
      | -0.00961416539377826	5.59949992625814	0.175411408314269
      | -0.00961390038512702	5.59950045392409	0.175409940322377
      | -0.00961355937737733	5.59950115284092	0.175408124271236
      | -0.00961305742513499	5.59950221082076	0.175405594713613
      | -0.00961248407606773	5.59950344686876	0.175402900140738
      | -0.00961136484811677	5.59950590175048	0.175398166952920
      | -0.00961075961331482	5.59950723853690	0.175395858791475
      | -0.00961050002658480	5.59950781230077	0.175394916813809
      | -0.00961043932705110	5.59950794645927	0.175394700485852
      | -0.00961035618584303	5.59950813020524	0.175394406546763
      | -0.00961026927607010	5.59950832225768	0.175394102174025
      | -0.00961016453412767	5.59950855367626	0.175393739215547
      | -0.00960991902004380	5.59950909589371	0.175392904618294
      | -0.00960874165475551	5.59951168880881	0.175389193470949
      | -0.00960649167138924	5.59951659437934	0.175383226831461
      | -0.00960382399913822	5.59952231514609	0.175377640503004
      | -0.00960131919537282	5.59952759933892	0.175373532171584
      | -0.00959811143930907	5.59953426240533	0.175369548332501
      | -0.00959737909930245	5.59953576959062	0.175368811593024
      | -0.00959714304227642	5.59953625440342	0.175368586687775
      | -0.00959704450892712	5.59953645663004	0.175368494585887
      | -0.00959664931016856	5.59953726690504	0.175368135560122
      | -0.00959610450454947	5.59953838182756	0.175367667349081
      | -0.00959529779128135	5.59954002847392	0.175367029242720
      | -0.00959485098449338	5.59954093839711	0.175366703315664
      | -0.00959426679106993	5.59954212596485	0.175366305866452
      | -0.00959370437466248	5.59954326706066	0.175365953196828
      | -0.00959317370214982	5.59954434185353	0.175365646706182
      | -0.00959287931142259	5.59954493732902	0.175365487458153
      | -0.00959259210663335	5.59954551775745	0.175365339391416
      | -0.00959213197301565	5.59954644664232	0.175365116971565
      | -0.00959174014636484	5.59954723666816	0.175364941712388
      | -0.00959160416280851	5.59954751064459	0.175364883888749
      | -0.00959146638781423	5.59954778812593	0.175364826866136
      | -0.00959126110168126	5.59954820138340	0.175364744801726
      | -0.00959117044820868	5.59954838380362	0.175364709660860
      | -0.00959104823793611	5.59954862965546	0.175364663346694
      | -0.00959023207490815	5.59955026954892	0.175364384838556
      | -0.00958868480163912	5.59955336954850	0.175363999478415
      | -0.00958586223783811	5.59955899860060	0.175363750240550
      | -0.00958250416374703	5.59956566054899	0.175364159817895
      | -0.00957634567656271	5.59957781126117	0.175366709133586
      | -0.00957431976565777	5.59958179631437	0.175368015679122
      | -0.00957210372796618	5.59958615148196	0.175369694509873
      | -0.00956835163218319	5.59959352075253	0.175373108667478
      | -0.00956300860515264	5.59960401622235	0.175379152153413
      | -0.00956078785093807	5.59960838252609	0.175382055834697
      | -0.00955898971850392	5.59961192070929	0.175384570704748
      | -0.00955824544265833	5.59961338608313	0.175385653967471
      | -0.00955771557310775	5.59961442965721	0.175386440150219
      | -0.00955596499530350	5.59961787955125	0.175389125481807
      | -0.00955285438588737	5.59962401876535	0.175394226059336
      | -0.00954797074651731	5.59963368479403	0.175403066720426
      | -0.00954121431264982	5.59964712319438	0.175416933615475
      | -0.00953168609703242	5.59966622560975	0.175439628342069
      | -0.00952190291778693	5.59968604338054	0.175466655261391
      | -0.00951844205476480	5.59969310581245	0.175477103688598
      | -0.00951538926711410	5.59969935817375	0.175486701040885
      | -0.00951145476775497	5.59970744753646	0.175499593357307
      | -0.00950847072073686	5.59971360591213	0.175509761447002
      | -0.00950523024100264	5.59972031571905	0.175521181830708
      | -0.00950023869792943	5.59973069530057	0.175539538299072
      | -0.00949807751616924	5.59973520534330	0.175547771425221
      | -0.00949338199415201	5.59974503592747	0.175566247625893
      | -0.00949068666779253	5.59975069765418	0.175577214133861
      | -0.00949016831177532	5.59975178800071	0.175579353107013
      | -0.00948910860067040	5.59975401853960	0.175583755870687
      | -0.00948600961065897	5.59976055242415	0.175596860515260
      | -0.00948506352860394	5.59976255027548	0.175600928888844
      | -0.00948414731188409	5.59976448640639	0.175604898835401
      | -0.00948138757354490	5.59977032592425	0.175617034040194
      | -0.00947474832690421	5.59978441723378	0.175647303698926
      | -0.00946844414083319	5.59979784401458	0.175677418523557
      | -0.00945920449736417	5.59981757931192	0.175723878430600
      | -0.00944850878752811	5.59984046060604	0.175780919769000
      | -0.00944638125139338	5.59984501137209	0.175792661154106
      | -0.00944553195392969	5.59984682763086	0.175797383463175
      | -0.00944287517531078	5.59985250740018	0.175812283426777
      | -0.00943249001813623	5.59987466541751	0.175872301515149
      | -0.00942381664007815	5.59989308756279	0.175924437862620
      | -0.00942284213290026	5.59989515120138	0.175930401989734
      | -0.00941855157672192	5.59990421953988	0.175956901457446
      | -0.00941230576738061	5.59991736438815	0.175996144367923
      | -0.00940411083470496	5.59993449656692	0.176048736483400
      | -0.00938950853889138	5.59996464942788	0.176145136941381
      | -0.00937423387211455	5.59999561224189	0.176248982357385
      | -0.00935526505470597	5.60003317911874	0.176381145043704
      | -0.00933585871092843	5.60007060050152	0.176518960894930
      | -0.00931604194979806	5.60010783179783	0.176661532302941
      | -0.00929011938151834	5.60015525966302	0.176849880350645
      | -0.00925959070233010	5.60020973265278	0.177073493097301
      | -0.00923348447063248	5.60025559171139	0.177265860702672
      | -0.00920334662176841	5.60030824447014	0.177488999416918
      | -0.00917034609517931	5.60036613599344	0.177734249517143
      | -0.00913314292760859	5.60043233420601	0.178010859302696
      | -0.00908685461442541	5.60051668882340	0.178352389112986
      | -0.00903744540809464	5.60060929147098	0.178709204400703
      | -0.00897844248698685	5.60072279474436	0.179120195701022
      | -0.00893181003313335	5.60081432045131	0.179433652812525
      | -0.00887061180691879	5.60093669818707	0.179835265242820
      | -0.00880480833167083	5.60107134262598	0.180264908945447
      | -0.00873606232590058	5.60121551074236	0.180723223748808
      | -0.00865879304025718	5.60138120875932	0.181260699522119
      | -0.00856942742410172	5.60157569878934	0.181918024213396
      | -0.00849169259632169	5.60174548821591	0.182519502896296
      | -0.00841110748955748	5.60192089283498	0.183166836436582
      | -0.00831377655997431	5.60213138610424	0.183971522387348
      | -0.00819432695481410	5.60238807696382	0.184976765715879
      | -0.00808536622146700	5.60262169450668	0.185895876034307
      | -0.00797022078811087	5.60286945189392	0.186858782487305
      | -0.00784592763057489	5.60313966566267	0.187886154395157
      | -0.00771710013792048	5.60342439107699	0.188946392213740
      | -0.00757242714409609	5.60375039248782	0.190152143246344
      | -0.00739368236927299	5.60415997162465	0.191697397777199
      | -0.00722242444236841	5.60455483891801	0.193254669006606
      | -0.00700129394090796	5.60506260665006	0.195367754195511
      | -0.00679471357068375	5.60553424356559	0.197412185458009
      | -0.00652464852565853	5.60615328216814	0.200138663987371
      | -0.00627420014055757	5.60673796158928	0.202720064289784
      | -0.00599996137449579	5.60739255363513	0.205664513599766
      | -0.00562641781177876	5.60829519610228	0.209990085775070
      | -0.00521696508895175	5.60928376051770	0.215168522503812
      | -0.00481934310500799	5.61025655847381	0.220612623453521
      | -0.00443954233141163	5.61121408297297	0.226354685446497
      | -0.00427072109836256	5.61164655120329	0.229158389261318
      | -0.00417745240670358	5.61188695912204	0.230813362448010
      | -0.00397342316243982	5.61242217700590	0.234783747264558
      | -0.00378757207055153	5.61293340688234	0.238906609982317
      | -0.00362714069969822	5.61340671216948	0.242941885451026
      | -0.00344922625824587	5.61397228524598	0.248100905825506
      | -0.00332198252103237	5.61439176401102	0.252396197469382
      | -0.00317380802312659	5.61488520996661	0.258430590524193
      | -0.00303972761239005	5.61536122766998	0.265963532406038
      | -0.00297112911350624	5.61566447767928	0.272412063375099
      | -0.00294177591821288	5.61588397421823	0.279637315919255
      | -0.00295415727756815	5.61596148523977	0.285645787514246
      | -0.00299926375668082	5.61594936956720	0.291413384787019
      | -0.00309741823084635	5.61582785100634	0.298460840063633
      | -0.00324579405697248	5.61557132003077	0.305847040208363
      | -0.00349085875552207	5.61507084304715	0.314818388567666
      | -0.00376774541096158	5.61446425187502	0.322755505892815
      | -0.00411426675726112	5.61366006942140	0.331130652599098
      | -0.00454244263652393	5.61261857572137	0.339947056189521
      | -0.00477258311955422	5.61204559745330	0.344201911041510
      | -0.00489677137307040	5.61173035229647	0.346389071758474
      | -0.00506918682023553	5.61129051134911	0.349282109761699
      | -0.00531205185014488	5.61067624903973	0.353073381893978
      | -0.00561336179414353	5.60993077450163	0.357394986347284
      | -0.00591302830061631	5.60920302294001	0.361417956696695
      | -0.00625206893937165	5.60837141824358	0.365827479789574
      | -0.00682030223965127	5.60691488876741	0.372985049943967
      | -0.00722032256794013	5.60585929901036	0.377716786209285
      | -0.00777255634309634	5.60439887961115	0.383896411878504
      | -0.00825848457022410	5.60309575872937	0.389092095181244
      | -0.00866894835375257	5.60199540863296	0.393221511516327
      | -0.00899419950485858	5.60112851788996	0.396374374676023
      | -0.00925988392717033	5.60044378945499	0.398736129310731
      | -0.00938580402196002	5.60015620049706	0.399696024819293
      | -0.00940465750619939	5.60012520927308	0.399781048875383
      | -0.00940872715100970	5.60012095914578	0.399787727353986
      | -0.00940956395322063	5.60012032893477	0.399787962210001
      | -0.00940980071568373	5.60012017084018	0.399787934893996
      | -0.00940987345644522	5.60012012420548	0.399787917533251
      | -0.00940989472287807	5.60012011074753	0.399787911642519
      | -0.00940989956826509	5.60012010769247	0.399787910248409
      | -0.00940990187966479	5.60012010623658	0.399787909576569
      | -0.00940990232104117	5.60012010595868	0.399787909447776
      | -0.00940990258814348	5.60012010579052	0.399787909369758
      | -0.00940990369761446	5.60012010509217	0.399787909045217
      | -0.00941008259656648	5.60011999557585	0.399787847228845
      | -0.00941244328677371	5.60011916647533	0.399785184560485
      | -0.00942015027637510	5.60012708347119	0.399746187509986
      | -0.00942460337370191	5.60015080269495	0.399676962801764
      | -0.00942457939309369	5.60018406619039	0.399615975681999
      | -0.00941939697003227	5.60020494386994	0.399630687510365
      | -0.00941809926148267	5.60020472198846	0.399642885284955
      | -0.00941809646464023	5.60020472011972	0.399642912893012
      | -0.00941809632166068	5.60020472002424	0.399642914304116
      | -0.00941809529264812	5.60020471933981	0.399642924447003
      | -0.00941809022536559	5.60020471603857	0.399642974073524
      | -0.00941805042241661	5.60020469374369	0.399643347040216
      | -0.00941722540525483	5.60020481269388	0.399648422908804
      | -0.00940354347280968	5.60021890460555	0.399677547760716
      | -0.00935356927480788	5.60028439414901	0.399721712851320
      | -0.00927071878154639	5.60040205356598	0.399768624187430
      | -0.00912582162411015	5.60061771674486	0.399851296108239
      | -0.00889009377171745	5.60097610335094	0.400016743928284
      | -0.00854404903172922	5.60150371934651	0.400296438985490
      | -0.00794083855814920	5.60242302254941	0.400782160189701
      | -0.00707971612176901	5.60373563885687	0.401443067798197
      | -0.00534456917415794	5.60634958653064	0.402846278851712
      | -0.00236193563805866	5.61071173080392	0.405281817891881
      | 0.000850696631445359	5.61523715643595	0.408000159735851
      | 0.00553114616947638	5.62153064455041	0.412048540656729
      | 0.0111702695649393	5.62868665338420	0.417125806243002
      | 0.0201522354392291	5.63925520131330	0.425593040930879
      | 0.0312534717025563	5.65111468313567	0.436698565663011
      | 0.0446692234428145	5.66394965589810	0.451065253068242
      | 0.0614285990067779	5.67801482341478	0.470467210669928
      | 0.0710026945492186	5.68516901862673	0.482285959484482
      | 0.102857777525894	5.70474790930640	0.525720875815169
      | 0.125980963350287	5.71499883264358	0.561616769806542
      | 0.155392618093574	5.72291812012597	0.613658625050095
      | 0.177976950099089	5.72446261281318	0.659742000404031
      | 0.186402738750261	5.72377531487644	0.678701619665102
      | 0.194467944371706	5.72237864310441	0.697874190502370
      | 0.204407681079298	5.71957566201060	0.723079356610694
      | 0.214713664755717	5.71509477919624	0.751602698860259
      | 0.228848108877095	5.70541567890370	0.796078172567560
      | 0.242128617399965	5.69068893392059	0.846604733098713
      | 0.251612191848604	5.67403581452523	0.892323634459026
      | 0.259836129324011	5.64955118227123	0.947940046380928
      | 0.263882176945330	5.62470632553446	0.995800377834735
      | 0.264967726315505	5.59867719163687	1.03976707486368
      | 0.263777526922292	5.57424460668383	1.07679436785427
      | 0.258187299477024	5.53391457696302	1.13108020730702
      | 0.252222755433260	5.50624549880072	1.16439041698426
      | 0.239252338785266	5.46054507127867	1.21375017906571
      | 0.209827636326645	5.38275407252943	1.28462756879173
      | 0.198844779385461	5.35805936501460	1.30417277710577
      | 0.179305728700449	5.31745981638084	1.33353530498301
      | 0.163395343937136	5.28667132704732	1.35361839781895
      | 0.151625942353265	5.26485172603345	1.36675141004773
      | 0.136517996272258	5.23772657339813	1.38182866353518
      | 0.128197645412688	5.22309420354035	1.38938813282132
      | 0.121138328147994	5.21069814325918	1.39544555515289
      | 0.114377897284350	5.19889805137106	1.40093888473157
      | 0.108910201044307	5.18944921083465	1.40516594306354
      | 0.102725623636542	5.17881959216186	1.40974147635205
      | 0.0968153521876527	5.16864006922043	1.41393239719250
      | 0.0880882408321413	5.15343804428655	1.41980314009736
      | 0.0799187539672176	5.13895120880123	1.42495964048483
      | 0.0729722645390773	5.12638713055599	1.42910422981357
      | 0.0649287129082879	5.11137867858187	1.43363889659150
      | 0.0581176912511976	5.09803263018636	1.43728004596201
      | 0.0530793288663017	5.08761786711194	1.43985600538600
      | 0.0472804116037149	5.07482436460723	1.44269846356170
      | 0.0413515855421865	5.06033884537032	1.44547877522109
      | 0.0380279922431712	5.05121537874385	1.44698353568940
      | 0.0341927780214817	5.03917963982955	1.44867175207393
      | 0.0322476174373783	5.03206314819844	1.44950830102023
      | 0.0299234511159822	5.02189893217722	1.45049154067430
      | 0.0292317703300223	5.01828405432480	1.45078056190210
      | 0.0283337660089480	5.01287427442704	1.45115406313427
      | 0.0275117744619565	5.00667052481381	1.45149261002180
      | 0.0271781540661641	5.00348665865758	1.45163010796231
      | 0.0269016933022727	5.00025276865334	1.45174362054416
      | 0.0267035521964729	4.99727875418338	1.45182509800265
      | 0.0265747877633298	4.99467947579532	1.45187884017010
      | 0.0264918827167583	4.99222900806491	1.45191373360617
      | 0.0264621197929348	4.99085030188924	1.45192701560690
      | 0.0264521776704090	4.99017745384235	1.45193189981945
      | 0.0264440779141770	4.98932182948222	1.45193643525504
      | 0.0264419395740808	4.98885905612665	1.45193805751633
      | 0.0264417033291652	4.98828462450875	1.45193930878641
      | 0.0264433269172072	4.98789239971919	1.45193976239199
      | 0.0264447600062157	4.98770243640168	1.45193988694503
      | 0.0264472726001939	4.98747076140755	1.45193995298330
      | 0.0264501370505296	4.98728851632471	1.45193991626425
      | 0.0264553595415671	4.98709308818403	1.45193971920212
      | 0.0264600038827567	4.98703736709415	1.45193956914603
      | 0.0264624464077312	4.98705081274874	1.45193913896024
      | 0.0264657066628763	4.98710395933750	1.45193786534315
      | 0.0264708409005285	4.98719979593902	1.45193574241001
      | 0.0264775128775781	4.98728670105683	1.45193451009271]
  Subsystem : Subsystem
  Transform : sm_lib/Frames and Transforms/Rigid Transform  TranslationMethod=Cartesian  TranslationStandardOffset=0  TranslationStandardOffsetUnits=m  TranslationStandardAxis=+Z  TranslationCartesianOffset=smiData.RigidTransform(13).translation  TranslationCartesianOffsetUnits=mm  TranslationROffset=0  TranslationROffsetUnits=m  TranslationZOffset=0  TranslationZOffsetUnits=m  TranslationThetaOffset=0  TranslationThetaOffsetUnits=deg  RotationMethod=ArbitraryAxis  RotationAngleUnits=rad  RotationStandardAxis=+Z  RotationAngle=smiData.RigidTransform(13).angle  RotationArbitraryAxis=smiData.RigidTransform(13).axis  FollAlignAxisA=+X  BaseAlignAxisA=+Y  FollAlignAxisB=+Y  BaseAlignAxisB=+Z  RotationSequenceAxes=FollowerAxes  RotationSequence=XYX  RotationSequenceAngles=[0 0 0]  RotationSequenceAnglesUnits=deg  RotationMatrix=[1 0 0; 0 1 0; 0 0 1]  Quaternion=[1 0 0 0]
  Transform1 : sm_lib/Frames and Transforms/Rigid Transform  TranslationMethod=None  TranslationStandardOffset=8  TranslationStandardOffsetUnits=mm  TranslationStandardAxis=+Y  TranslationCartesianOffset=[20000 0 0]  TranslationCartesianOffsetUnits=mm  TranslationROffset=0  TranslationROffsetUnits=m  TranslationZOffset=0  TranslationZOffsetUnits=m  TranslationThetaOffset=0  TranslationThetaOffsetUnits=deg  RotationMethod=StandardAxis  RotationAngleUnits=deg  RotationStandardAxis=-X  RotationAngle=90  RotationArbitraryAxis=robotData.RigidTransform(29).axis  FollAlignAxisA=+X  BaseAlignAxisA=+Y  FollAlignAxisB=+Y  BaseAlignAxisB=+Z  RotationSequenceAxes=FollowerAxes  RotationSequence=XYX  RotationSequenceAngles=[0 0 0]  RotationSequenceAnglesUnits=deg  RotationMatrix=[1 0 0; 0 1 0; 0 0 1]  Quaternion=[1 0 0 0]
  Weld Joint : sm_lib/Joints/Weld Joint  JointMode=Normal  SenseConstraintForce=off  SenseConstraintForceX=off  SenseConstraintForceY=off  SenseConstraintForceZ=off  SenseConstraintTorque=off  SenseConstraintTorqueX=off  SenseConstraintTorqueY=off  SenseConstraintTorqueZ=off  SenseTotalForce=off  SenseTotalForceX=off  SenseTotalForceY=off  SenseTotalForceZ=off  SenseTotalTorque=off  SenseTotalTorqueX=off  SenseTotalTorqueY=off  SenseTotalTorqueZ=off  CompositeWrenchDir=FollowerOnBase  CompositeWrenchFrame=BaseFrame
  Weld Joint1 : sm_lib/Joints/Weld Joint  JointMode=Normal  SenseConstraintForce=off  SenseConstraintForceX=off  SenseConstraintForceY=off  SenseConstraintForceZ=off  SenseConstraintTorque=off  SenseConstraintTorqueX=off  SenseConstraintTorqueY=off  SenseConstraintTorqueZ=off  SenseTotalForce=off  SenseTotalForceX=off  SenseTotalForceY=off  SenseTotalForceZ=off  SenseTotalTorque=off  SenseTotalTorqueX=off  SenseTotalTorqueY=off  SenseTotalTorqueZ=off  CompositeWrenchDir=FollowerOnBase  CompositeWrenchFrame=BaseFrame
  World : sm_lib/Frames and Transforms/World Frame
  Ground contact : PMIOPort  Side=Right
  World Ref : PMIOPort  Port=2  Side=Right
  Base Ref : PMIOPort  Port=3  Side=Right
  Platform stop Threshold : Outport
  Platform xy : Outport  Port=2
  Theta platform : Outport  Port=3
  wires:
  Control/2(Right_Trq) -> Simulink-PS Converter1/1
  PS-Simulink Converter1/1 -> Product/2, Actuation velocity/1
  PS-Simulink Converter2/1 -> Bus Creator/2  "R"
  PS-Simulink Converter/1 -> Product/1, Actuation torque/1
  Base_1_RIGID/1(Measure) -> Control/2(Measure)
  PS-Simulink Converter3/1 -> Bus Creator/1  "L"
  Bus Creator/1 -> Control/1(wheel)
  Platform waypoints/1 -> Control/3(Platform waypoints)
  Control/3(stopThreshold) -> Platform stop Threshold/1
  Control/4(Platform xy) -> Platform xy/1
  PS-Simulink Converter4/1 -> Actuation torque/2
  Control/1(Left_Trq) -> Scope2/1, Scope/1, Simulink-PS Converter2/1
  Subsystem/1(Out1) -> Scope1/1
  platform_mode_out/1 -> Control/4("platform_mode_out ")
  Base_1_RIGID/2(Theta Platfrom) -> Theta platform/1
  Product/1 -> Power/1
  connections:
  Caster_coupler_1_RIGID/LConn1 -- Revolute/RConn1
  Battery/RConn1 -- Electrical Reference/LConn1 -- Connection Label/LConn1
  Bushing Joint/LConn1 -- Transform/RConn1
  PS Terminator1/LConn1 -- Motor & Drive (System Level)1/RConn2
  Rotational Multibody Interface/LConn2 -- Motor & Drive (System Level)1/RConn3 -- Mechanical Rotational Reference/LConn1
  Weld Joint1/RConn1 -- Coupler_1_RIGID/LConn1
  Weld Joint/LConn1 -- Base_1_RIGID/RConn2
  Connection Label5/LConn1 -- Motor & Drive (System Level)1/RConn1
  Motor & Drive (System Level)1/LConn3 -- Gear Box/LConn1
  Coupler_2_RIGID/RConn1 -- Revolute3/RConn1
  PS Terminator/LConn1 -- Motor & Drive (System Level)/RConn2
  Ground contact/RConn1 -- Spatial Contact Force2/LConn1 -- Spatial Contact Force4/LConn1 -- Spatial Contact Force3/LConn1
  Rotational Multibody Interface1/LConn1 -- Revolute3/LConn2
  Connection Label2/LConn1 -- Motor & Drive (System Level)/LConn1
  Base_1_RIGID/LConn2 -- Cam/LConn1 -- Bushing Joint/RConn1
  Revolute2/RConn2 -- PS-Simulink Converter1/LConn1 -- PS-Simulink Converter3/LConn1 -- Rotational Multibody Interface/RConn1
  Revolute2/RConn3 -- PS-Simulink Converter/LConn1
  Coupler_1_RIGID/RConn1 -- Revolute2/RConn1
  Revolute3/RConn2 -- PS-Simulink Converter2/LConn1 -- Rotational Multibody Interface1/RConn1
  Caster_coupler_1_RIGID/RConn1 -- Revolute1/LConn1
  Gear Box2/RConn1 -- Rotational Multibody Interface1/RConn2
  Left Wheel/RConn1 -- Revolute2/LConn1
  Simulink-PS Converter2/RConn1 -- Motor & Drive (System Level)1/LConn2
  Rigid Transform1/RConn1 -- Transform/LConn1
  Weld Joint/RConn1 -- Coupler_2_RIGID/LConn1
  Revolute1/RConn1 -- Small Wheel/LConn1
  Connection Label3/LConn1 -- Motor & Drive (System Level)/RConn1
  Right Wheel/RConn1 -- Revolute3/LConn1
  Rotational Multibody Interface1/LConn2 -- Mechanical Rotational Reference1/LConn1 -- Motor & Drive (System Level)/RConn3
  Spatial Contact Force3/RConn1 -- Left Wheel/LConn1
  Connection Label4/LConn1 -- Motor & Drive (System Level)1/LConn1
  Camera Position/RConn1 -- Cam/RConn1
  Rotational Multibody Interface/LConn1 -- Revolute2/LConn2 -- PS-Simulink Converter4/LConn1
  Base_1_RIGID/RConn1 -- Revolute/LConn1
  Simulink-PS Converter1/RConn1 -- Motor & Drive (System Level)/LConn2
  Connection Label1/LConn1 -- Battery/LConn1
  Base_1_RIGID/LConn1 -- Weld Joint1/LConn1
  Base_1_RIGID/RConn3 -- Transform1/LConn1
  Base Ref/RConn1 -- Transform1/RConn1
  MechanismConfiguration/RConn1 -- Spline/LConn1 -- Point Cloud/LConn1 -- Point Cloud1/LConn1 -- World/RConn1 -- World Ref/RConn1 -- Rigid Transform1/LConn1 -- Solver Configuration/RConn1
  Left Wheel/RConn2 -- Subsystem/RConn1
  Right Wheel/RConn2 -- Subsystem/RConn2
  Spatial Contact Force4/RConn1 -- Small Wheel/RConn1
  Spatial Contact Force2/RConn1 -- Right Wheel/LConn1
  Gear Box/RConn1 -- Rotational Multibody Interface/RConn2
  Gear Box2/LConn1 -- Motor & Drive (System Level)/LConn3
